simulink subsystem "EncoderAJ_Velocidad"  (R2023b)
settings: Solver=VariableStepAuto  StartTime=0.0  StopTime=10.0  RelTol=1e-3
libraries: arduinosensorlib x2, simulink x1
settings Model: Creator=marqu  LastModifiedBy=marqu

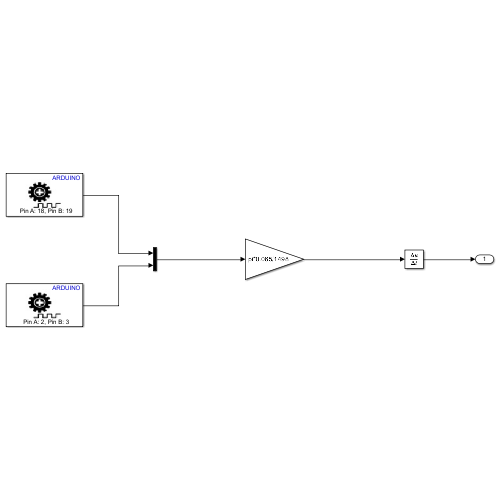
[thumbnail: Simulink's stored preview of the top-level diagram]
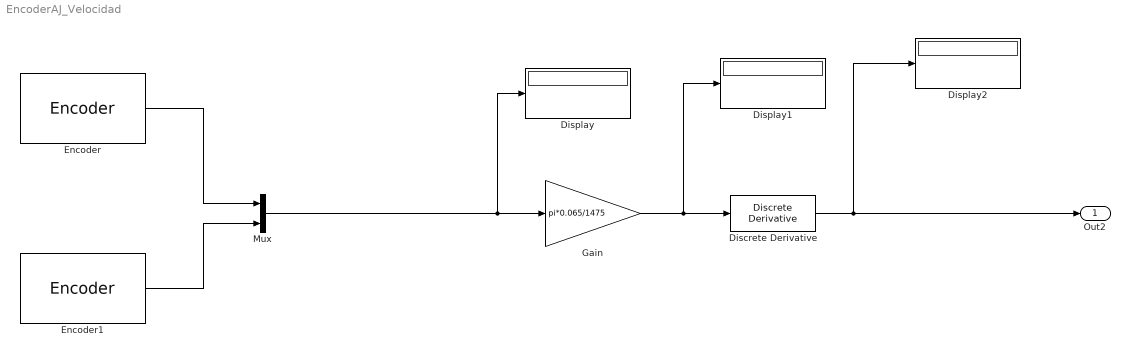
== system EncoderAJ_Velocidad ==
  Discrete Derivative : simulink/Discrete/Discrete Derivative  gainval=1.0  ICPrevScaledInput=0.0  OutMin=[]  OutMax=[]  OutDataType=fixdt(1, 16)  OutScaling=2^-10  DoSatur=off
  Display : Display
  Display1 : Display
  Display2 : Display
  Encoder : arduinosensorlib/Encoder  InputA=18  InputB=19  Mode=No reset  SampleTime=-1
  Encoder1 : arduinosensorlib/Encoder  InputA=2  InputB=3  Mode=No reset  SampleTime=-1
  Gain : Gain  Gain=pi*0.065/1475  OutDataTypeStr=double
  Mux : Mux  Inputs=2
  Out2 : Outport
  wires:
  Encoder1/1 -> Mux/2
  Encoder/1 -> Mux/1
  Gain/1 -> Display1/1, Discrete Derivative/1
  Mux/1 -> Gain/1, Display/1
  Discrete Derivative/1 -> Out2/1, Display2/1
